simulink model "Sim_Inverse_kinematics"  (R2019a)
settings: Solver=VariableStepAuto  StartTime=0.0  StopTime=10  RelTol=1e-3
libraries: robotcorelib x1, robotmaniplib x1, vrlib x1
settings Model: Creator=rajeshree  LastModifiedBy=rajeshree

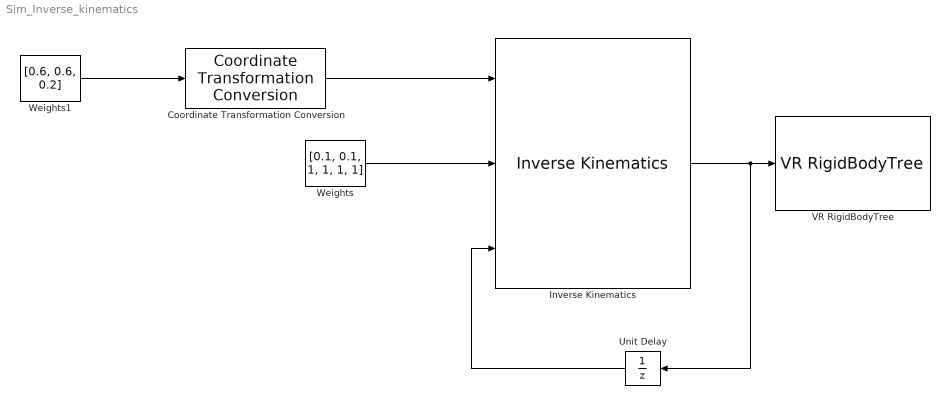
== system Sim_Inverse_kinematics ==
  Coordinate Transformation Conversion : robotcorelib/Coordinate Transformation Conversion  InputRepresentation=Translation Vector  InputEulerSequence=ZYX  ShowTrVecInputPort=on  OutputRepresentation=Homogeneous Transformation  OutputEulerSequence=ZYX  ShowTrVecOutputPort=on  SimulateUsing=Interpreted execution
      settings: SourceProductBaseCode=RO
  Inverse Kinematics : robotmaniplib/Inverse Kinematics  RigidBodyTree=newSubtree  EndEffector=r_hand  ShowInfo=off  SolverName=BFGS Gradient Projection  EnforceJointLimits=on  MaxIterations=1500  MaxTime=10  GradientTolerance=1e-7  SolutionTolerance=1e-6  StepTolerance=1e-14  ErrorChangeTolerance=1e-12  UseErrorDamping=on  DampingBias=0.0025  SimulateUsing=Interpreted execution
      settings: SourceProductName=Robotics System Toolbox
  Unit Delay : UnitDelay  InitialCondition=zeros(7,1)  SampleTime=-1  HasFrameUpgradeWarning=on
  VR RigidBodyTree : vrlib/VR RigidBodyTree  VrmlFile=/home/rajeshree/catkin_ws/src/Dual-Arm-Manipulation/atlas.wrl  RBT=newSubtree  useRBT=on  Ts=-1  ForceViewerOpen=on
      settings: SourceProductName=Simulink  SourceProductBaseCode=SL
  Weights : Constant  Value=[0.1, 0.1, 1, 1, 1, 1]
  Weights1 : Constant  Value=[0.6, 0.6, 0.2]
  wires:
  Inverse Kinematics/1 -> Unit Delay/1, VR RigidBodyTree/1
  Weights/1 -> Inverse Kinematics/2
  Coordinate Transformation Conversion/1 -> Inverse Kinematics/1
  Weights1/1 -> Coordinate Transformation Conversion/1
  Unit Delay/1 -> Inverse Kinematics/3
